simulink library "lib_energy_storage2"  (Simulink 4.1.1)
values from neighbouring files (symbols this model uses):
  logFlag = 1    [advSACompMaskInit.m]    (also in advSACompMaskInitR13.m)
undefined symbols (not defined in the file or in its folder): air_cp, amb_tmp, cyc_mph, enable_stop, ess_cap_scale, ess_cb, ess_cc, ess_coulombic_eff, ess_init_soc, ess_max_ah_cap, ess_max_p, ess_max_p_soc, ess_max_soc, ess_max_volts, ess_min_soc, ess_min_volts, ess_MMi, ess_MMo, ess_mod_airflow, ess_mod_cp, ess_mod_cpm, ess_mod_init_tmp, ess_module_mass, ess_module_num, ess_on, ess_parallel_mod_num, ess_res_scale_coef, ess_res_scale_fun, ess_set_tmp, ess_soc, ess_th_calc, ess_th_res, ess_th_res_off, ess_th_res_on, ess_tmp, ess_voc, fund_byu, fund_byuop, mc_min_volts, saber_air_temp, Saber_Battery_IO_File, saber_init_soc, saber_init_temp, saber_init_voc, saber_k_cb, saber_k_cc, saber_k_rc, saber_k_re, saber_k_rt, saber_k_soc, t_soc, time_step
libraries: simulink3 x16, lib_energy_storage x1, lib_energy_storage2 x1
(part 10 of 10)

== system lib_energy_storage2/energy storage <ess> nnet/energy storage <ess> nnet/model/NNet/Neural Network/Layer 2/LW{2,1} ==
  "ad{2,1}" : Inport  Port=1  LatchInput=off  PortDimensions=3
  "IW{2,1}(1,:)'" : Constant  Value=[-0.2776092;-2.6799360000000001;-2.2138360000000001]
      mask Display: disp('weights')
  "IW{2,1}(2,:)'" : Constant  Value=[3.601111;2.064257;0.86618079999999997]
      mask Display: disp('weights')
  Mux : Mux  Inputs=2
      settings: DisplayOption=none
  dotprod1 : Subsystem
      settings: RTWFcnNameOpts=Auto  RTWFileNameOpts=Auto
  dotprod2 : Subsystem
      settings: RTWFcnNameOpts=Auto  RTWFileNameOpts=Auto
  "lz{2,1}" : Outport  Port=1  InitialOutput=0
  wires:
  Mux/1 -> "lz{2,1}"/1
  dotprod2/1(z) -> Mux/2
  "ad{2,1}"/1 -> dotprod2/2(p), dotprod1/2(p)
  "IW{2,1}(2,:)'"/1 -> dotprod2/1(w)
  dotprod1/1(z) -> Mux/1
  "IW{2,1}(1,:)'"/1 -> dotprod1/1(w)

== system lib_energy_storage2/energy storage <ess> nnet/energy storage <ess> nnet/model/NNet/Neural Network/Layer 2/logsig ==
  n : Inport  Port=1  LatchInput=off
  Exp : ElementaryMath  Operator=exp
  Gain : Gain  Gain=-1  Multiplication=Element-wise(K.*u)  SaturateOnIntegerOverflow=on
  Reciprocal : ElementaryMath  Operator=reciprocal
  Sum : Sum  Inputs=++  SaturateOnIntegerOverflow=on
  one : Constant  Value=1
  a : Outport  Port=1  InitialOutput=0
  wires:
  n/1 -> Gain/1
  Gain/1 -> Exp/1
  Exp/1 -> Sum/1
  one/1 -> Sum/2
  Sum/1 -> Reciprocal/1
  Reciprocal/1 -> a/1

== system lib_energy_storage2/energy storage <ess> nnet/energy storage <ess> nnet/model/NNet/Neural Network/Layer 1/IW{1,1}/dotprod1 ==
  w : Inport  Port=1  LatchInput=off
  p : Inport  Port=2  LatchInput=off
  Dot Product : Subsystem  mask(Dot Product){}
      mask help:
      | Inner (dot) product.
      | y=sum(u1.*u2)
      mask init:
      | t=(0:.1:2*pi)';
      | x=cos(t);
      | y=sin(t);
      settings: RTWFcnNameOpts=Auto  RTWFileNameOpts=Auto
      mask Help: Computes the inner (dot) product of the inputs: sum(u1.*u2).  The inputs are vectors of the same length. Output is a scalar.
      mask Display: plot(0,0,1,1,x*[0.025 0.07]+0.5,y*[0.025 0.07]+0.5)
  z : Outport  Port=1  InitialOutput=0
  wires:
  w/1 -> Dot Product/1(in_1)
  p/1 -> Dot Product/2(in_2)
  Dot Product/1(out_1) -> z/1

== system lib_energy_storage2/energy storage <ess> nnet/energy storage <ess> nnet/model/NNet/Neural Network/Layer 1/IW{1,1}/dotprod2 ==
  w : Inport  Port=1  LatchInput=off
  p : Inport  Port=2  LatchInput=off
  Dot Product : Subsystem  mask(Dot Product){}
      mask help:
      | Inner (dot) product.
      | y=sum(u1.*u2)
      mask init:
      | t=(0:.1:2*pi)';
      | x=cos(t);
      | y=sin(t);
      settings: RTWFcnNameOpts=Auto  RTWFileNameOpts=Auto
      mask Help: Computes the inner (dot) product of the inputs: sum(u1.*u2).  The inputs are vectors of the same length. Output is a scalar.
      mask Display: plot(0,0,1,1,x*[0.025 0.07]+0.5,y*[0.025 0.07]+0.5)
  z : Outport  Port=1  InitialOutput=0
  wires:
  w/1 -> Dot Product/1(in_1)
  p/1 -> Dot Product/2(in_2)
  Dot Product/1(out_1) -> z/1

== system lib_energy_storage2/energy storage <ess> nnet/energy storage <ess> nnet/model/NNet/Neural Network/Layer 1/IW{1,1}/dotprod3 ==
  w : Inport  Port=1  LatchInput=off
  p : Inport  Port=2  LatchInput=off
  Dot Product : Subsystem  mask(Dot Product){}
      mask help:
      | Inner (dot) product.
      | y=sum(u1.*u2)
      mask init:
      | t=(0:.1:2*pi)';
      | x=cos(t);
      | y=sin(t);
      settings: RTWFcnNameOpts=Auto  RTWFileNameOpts=Auto
      mask Help: Computes the inner (dot) product of the inputs: sum(u1.*u2).  The inputs are vectors of the same length. Output is a scalar.
      mask Display: plot(0,0,1,1,x*[0.025 0.07]+0.5,y*[0.025 0.07]+0.5)
  z : Outport  Port=1  InitialOutput=0
  wires:
  w/1 -> Dot Product/1(in_1)
  p/1 -> Dot Product/2(in_2)
  Dot Product/1(out_1) -> z/1

== system lib_energy_storage2/energy storage <ess> nnet/energy storage <ess> nnet/model/NNet/Neural Network/Layer 2/LW{2,1}/dotprod1 ==
  w : Inport  Port=1  LatchInput=off
  p : Inport  Port=2  LatchInput=off
  Dot Product : Subsystem  mask(Dot Product){}
      mask help:
      | Inner (dot) product.
      | y=sum(u1.*u2)
      mask init:
      | t=(0:.1:2*pi)';
      | x=cos(t);
      | y=sin(t);
      settings: RTWFcnNameOpts=Auto  RTWFileNameOpts=Auto
      mask Help: Computes the inner (dot) product of the inputs: sum(u1.*u2).  The inputs are vectors of the same length. Output is a scalar.
      mask Display: plot(0,0,1,1,x*[0.025 0.07]+0.5,y*[0.025 0.07]+0.5)
  z : Outport  Port=1  InitialOutput=0
  wires:
  w/1 -> Dot Product/1(in_1)
  p/1 -> Dot Product/2(in_2)
  Dot Product/1(out_1) -> z/1

== system lib_energy_storage2/energy storage <ess> nnet/energy storage <ess> nnet/model/NNet/Neural Network/Layer 2/LW{2,1}/dotprod2 ==
  w : Inport  Port=1  LatchInput=off
  p : Inport  Port=2  LatchInput=off
  Dot Product : Subsystem  mask(Dot Product){}
      mask help:
      | Inner (dot) product.
      | y=sum(u1.*u2)
      mask init:
      | t=(0:.1:2*pi)';
      | x=cos(t);
      | y=sin(t);
      settings: RTWFcnNameOpts=Auto  RTWFileNameOpts=Auto
      mask Help: Computes the inner (dot) product of the inputs: sum(u1.*u2).  The inputs are vectors of the same length. Output is a scalar.
      mask Display: plot(0,0,1,1,x*[0.025 0.07]+0.5,y*[0.025 0.07]+0.5)
  z : Outport  Port=1  InitialOutput=0
  wires:
  w/1 -> Dot Product/1(in_1)
  p/1 -> Dot Product/2(in_2)
  Dot Product/1(out_1) -> z/1

== system lib_energy_storage2/energy storage <ess> nnet/energy storage <ess> nnet/model/NNet/Neural Network/Layer 1/IW{1,1}/dotprod1/Dot Product ==
  in_1 : Inport  Port=1  LatchInput=off
  in_2 : Inport  Port=2  LatchInput=off
  Product : Product  Inputs=2  Multiplication=Element-wise(.*)  SaturateOnIntegerOverflow=on
  Sum : Sum  Inputs=+  SaturateOnIntegerOverflow=on
  out_1 : Outport  Port=1  InitialOutput=0
  wires:
  in_2/1 -> Product/2
  in_1/1 -> Product/1
  Product/1 -> Sum/1
  Sum/1 -> out_1/1

== system lib_energy_storage2/energy storage <ess> nnet/energy storage <ess> nnet/model/NNet/Neural Network/Layer 1/IW{1,1}/dotprod2/Dot Product ==
  in_1 : Inport  Port=1  LatchInput=off
  in_2 : Inport  Port=2  LatchInput=off
  Product : Product  Inputs=2  Multiplication=Element-wise(.*)  SaturateOnIntegerOverflow=on
  Sum : Sum  Inputs=+  SaturateOnIntegerOverflow=on
  out_1 : Outport  Port=1  InitialOutput=0
  wires:
  in_2/1 -> Product/2
  in_1/1 -> Product/1
  Product/1 -> Sum/1
  Sum/1 -> out_1/1

== system lib_energy_storage2/energy storage <ess> nnet/energy storage <ess> nnet/model/NNet/Neural Network/Layer 1/IW{1,1}/dotprod3/Dot Product ==
  in_1 : Inport  Port=1  LatchInput=off
  in_2 : Inport  Port=2  LatchInput=off
  Product : Product  Inputs=2  Multiplication=Element-wise(.*)  SaturateOnIntegerOverflow=on
  Sum : Sum  Inputs=+  SaturateOnIntegerOverflow=on
  out_1 : Outport  Port=1  InitialOutput=0
  wires:
  in_2/1 -> Product/2
  in_1/1 -> Product/1
  Product/1 -> Sum/1
  Sum/1 -> out_1/1

== system lib_energy_storage2/energy storage <ess> nnet/energy storage <ess> nnet/model/NNet/Neural Network/Layer 2/LW{2,1}/dotprod1/Dot Product ==
  in_1 : Inport  Port=1  LatchInput=off
  in_2 : Inport  Port=2  LatchInput=off
  Product : Product  Inputs=2  Multiplication=Element-wise(.*)  SaturateOnIntegerOverflow=on
  Sum : Sum  Inputs=+  SaturateOnIntegerOverflow=on
  out_1 : Outport  Port=1  InitialOutput=0
  wires:
  in_2/1 -> Product/2
  in_1/1 -> Product/1
  Product/1 -> Sum/1
  Sum/1 -> out_1/1

== system lib_energy_storage2/energy storage <ess> nnet/energy storage <ess> nnet/model/NNet/Neural Network/Layer 2/LW{2,1}/dotprod2/Dot Product ==
  in_1 : Inport  Port=1  LatchInput=off
  in_2 : Inport  Port=2  LatchInput=off
  Product : Product  Inputs=2  Multiplication=Element-wise(.*)  SaturateOnIntegerOverflow=on
  Sum : Sum  Inputs=+  SaturateOnIntegerOverflow=on
  out_1 : Outport  Port=1  InitialOutput=0
  wires:
  in_2/1 -> Product/2
  in_1/1 -> Product/1
  Product/1 -> Sum/1
  Sum/1 -> out_1/1
